simulink model "zynqRadioWalkieTalkieRxAD9361AD9364SL"  (R2016a)
settings: Solver=ode45  StartTime=0.0  StopTime=inf  RelTol=1e-3
PostLoadFcn:
  | sdrzWalkieTalkieRxParams = zynqRadioWalkieTalkeRxHelperAD9361AD9364SL_SimParams;
  | sdrzWalkieTalkieRxHelper_ModelParamsMask('applyParametersToModel');
InitFcn:
  | sdrzWalkieTalkieRxParams = zynqRadioWalkieTalkeRxHelperAD9361AD9364SL_SimParams;
  | sdrzWalkieTalkieRxHelper_ModelParamsMask('applyParametersToModel');
undefined symbols (not defined in the file or in its folder): F, fdesignblkfcn, gcbh
libraries: dspsnks4 x1, sdrzblksprivate x1, zc706fmc234_lib x1, dspmlti4 x1, commrfcorlib x1
CloseFcn:
  | clear sdrzWalkieTalkieRxParams GoertzelCoeffs
Description:
  | This model uses Simulink(R) to receive an FM signal from a suitable commercial walkie-talkie using SDR hardware with Analog Devices FMCOMMS2/3/4.
settings Model: SimulationMode=accelerator  Creator=The MathWorks, Inc.  LastModifiedBy=The MathWorks, Inc.
settings DataIOCC: LimitDataPoints=on  SaveFormat=Array
settings DebuggingCC: SolverPrmCheckMsg=warning  ParameterPrecisionLossMsg=none  AllowSymbolicDim=off
settings HardwareCC: ProdBitPerPointer=32  ProdLargestAtomicFloat=None  ProdIntDivRoundTo=Undefined  ProdEndianess=Unspecified  ProdWordSize=32  ProdHWDeviceType=32-bit Generic
settings ModelReferenceCC: PropagateSignalLabelsOutOfModel=off
settings ConfigComp: CovModelRefEnable=Off  CovSFcnEnable=off

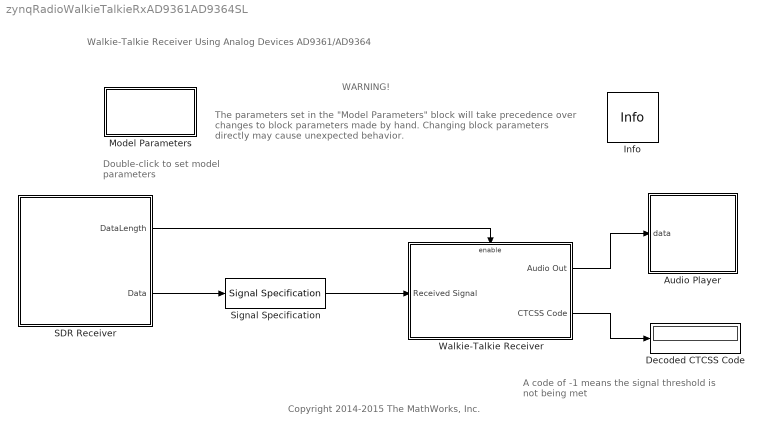
== system zynqRadioWalkieTalkieRxAD9361AD9364SL ==
  note: A code of -1 means the signal threshold
      | is not being met
  note: Walkie-Talkie Receiver Using Analog Devices AD9361/AD9364
  note: Double-click to
      | set model parameters
  note: The parameters set in the "Model Parameters" block will
      | take precedence over changes to block parameters made by hand.
      | Changing block parameters directly may cause unexpected behavior.
  note: WARNING!
  note: Copyright 2014-2015 The MathWorks, Inc.
  Audio Player : Subsystem
  Decoded CTCSS Code : Display
  Info : sdrzblksprivate/Info  SystemSampleTime=-1
  Model Parameters : Subsystem  TreatAsAtomicUnit=on  mask(Model Parameters){walkieTalkieProtocol=FRS, channelFRS=1, channelPMR446=4, CTCSSCode=5, CTCSSDecodeBlockLength=4000, signalPowerThreshold=0.1}
      mask prompts: walkieTalkieProtocol "Walkie-talkie protocol:"; channelFRS "Channel (1 to 14):"; channelPMR446 "Channel (1 to 8):"; CTCSSCode "CTCSS code (0 to 38):"; CTCSSDecodeBlockLength "CTCSS decode block length:"; signalPowerThreshold "Signal threshold for squelch:"
      mask help: Changing these values defines the model parameters needed for reception.
      mask init:
      | sdrzWalkieTalkieRxHelper_ModelParamsMask('applyParametersToModel');
      mask Help: sdrzdemohelp;
      mask TypeOptions walkieTalkieProtocol: FRS | PMR446
      mask Callback walkieTalkieProtocol: sdrzWalkieTalkieRxHelper_ModelParamsMask('maskDisplayUpdate');
      mask Display: disp('Model\nParameters');
  SDR Receiver : Subsystem
  Signal Specification : SignalSpecification  SampleTime=sdrzWalkieTalkieRxParams.radioFrameSize/sdrzWalkieTalkieRxParams.radioSampleRate
  Walkie-Talkie Receiver : Subsystem
  wires:
  Walkie-Talkie Receiver/2(CTCSS Code) -> Decoded CTCSS Code/1
  SDR Receiver/1(DataLength) -> Walkie-Talkie Receiver/Enable
  Walkie-Talkie Receiver/1(Audio Out) -> Audio Player/1(data)
  SDR Receiver/2(Data) -> Signal Specification/1
  Signal Specification/1 -> Walkie-Talkie Receiver/1(Received Signal)

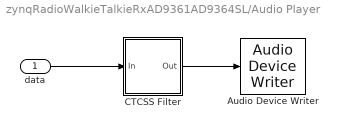
== system zynqRadioWalkieTalkieRxAD9361AD9364SL/Audio Player ==
  data : Inport
  Audio Device Writer : dspsnks4/Audio Device Writer  Driver=DirectSound  Device=Default  InheritSampleRate=off  SampleRate=8e3  BitDepth=16-bit integer  BufferSize=4096  NumBuffers=10  DefaultOutputChannelMapping=on  OutputChannelMapping=1:2  OutputNumUnderrunSamples=off  DriverIdx=1  DeviceWarnFlag=''
  CTCSS Filter : Subsystem  DialogController=fdesignblkfcn  InitFcn=fdesignblkfcn(gcbh, {'InitFcn'});  mask(Highpass Filter){}
      mask help: Design a highpass filter
      settings: CopyFcn=fdesignblkfcn(gcbh, {'CopyFcn'});
      mask Help: helpview(mapfilelocation('dsp'), 'dsphighpassfilter');
      mask Display: disp('Highpass')
  wires:
  data/1 -> CTCSS Filter/1(In)
  CTCSS Filter/1(Out) -> Audio Device Writer/1

== system zynqRadioWalkieTalkieRxAD9361AD9364SL/Model Parameters ==
  note: This subsystem is empty.
      | It is used for setting parameter values (in the mask).

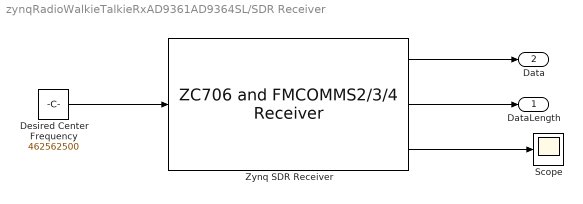
== system zynqRadioWalkieTalkieRxAD9361AD9364SL/SDR Receiver ==
  Desired Center Frequency : Constant  Value=462562500
  Scope : Scope
  Zynq SDR Receiver : zc706fmc234_lib/ZC706 and  FMCOMMS2//3//4  Receiver  IPAddress=192.168.3.2  CenterFrequencySource=Input port  CenterFrequency=2400000000  GainSource=AGC Fast Attack  Gain=1  ChannelMapping=1  BasebandSampleRate=sdrzWalkieTalkieRxParams.radioSampleRate  EnableBurstMode=off  NumFramesInBurst=20  OutputDataType=single  SamplesPerFrame=sdrzWalkieTalkieRxParams.radioFrameSize  LostSamplesOutputPort=on  RSSIOutputPort=off  DMATimeoutValue=1  blockMode=Normal  EnableQuadratureTracking=on  EnableRFDCTracking=on  EnableBasebandDCTracking=on  BypassUserLogic=on  ShowAdvancedProperties=on  ShowInternalProperties=off  subDeviceList=zynqReceiver  sdrExecutionMode=HW  dataUDPPort=-1  ctrlUDPPort=-1  SourceSelect=RF data  SourceConfiguration1=1023  FIRCoefficientSize=[ 128; 128 ]  FIRCoefficients=[ 111, -87, 147, -127, -18, -286, -312, -555, -601, -722, -642, -555, -303, -66, 221, 393, 488, 403, 219, -74, -343, -550, -582, -450, -146, 221, 569, 759, 735, 463, 20, -487, -885, -1048, -883, -418, 243, 897, 1340, 1394, 1002, 228, -715, -1549, -1980, -1819, -1028, 217, 1583, 2635, 2980, 2377, 853, -1275, -3435, -4926, -5080, -3454, 40, 5065, 10903, 16581, 21085, 23573, 23573, 21085, 16581, 10903, 5065, 40, -3454, -5080, -4926, -3435, -1275, 853, 2377, 2980, 2635, 1583, 217, -1028, -1819, -1980, -1549, -715, 228, 1002, 1394, 1340, 897, 243, -418, -883, -1048, -885, -487, 20, 463, 735, 759, 569, 221, -146, -450, -582, -550, -343, -74, 219, 403, 488, 393, 221, -66, -303, -555, -642, -722, -601, -555, -312, -286, -18, -127, 147, -87, 111; 382, -200, 711, -41, 645, 36, 346, -194, -119, -543, -472, -646, -404, -312, 45, 197, 413, 346, 241, -93, -373, -680, -755, -689, -356, 51, 515, 795, 870, 609, 136, -488, -1009, -1303, -1191, -712, 69, 885, 1516, 1692, 1336, 468, -662, -1740, -2378, -2329, -1494, -55, 1620, 2995, 3584, 3045, 1368, -1121, -3755, -5708, -6156, -4542, -710, 4969, 11669, 18243, 23486, 26391, 26391, 23486, 18243, 11669, 4969, -710, -4542, -6156, -5708, -3755, -1121, 1368, 3045, 3584, 2995, 1620, -55, -1494, -2329, -2378, -1740, -662, 468, 1336, 1692, 1516, 885, 69, -712, -1191, -1303, -1009, -488, 136, 609, 870, 795, 515, 51, -356, -689, -755, -680, -373, -93, 241, 346, 413, 197, 45, -312, -404, -646, -472, -543, -119, -194, 346, 36, 645, -41, 711, -200, 382 ]  FIRGain=[ 0; -12 ]  FIRDecimInterpFactor=[ 4; 4 ]  AnalogFilterCutoff=[ 2560000; 2560000 ]  FilterPathRates=[ 737280000, 184320000, 61440000, 30720000, 15360000, 3840000; 737280000, 184320000, 61440000, 30720000, 15360000, 3840000 ]  FilterDesignTypeForTx=DefaultFilterFromOther  FilterDesignTypeForRx=DefaultFilter  BISTLoopbackConfig=No Loopback  BISTPRBSMode=PRBS Disable  BISTToneMode=Tone Disable  BISTToneFrequency=F/32  BISTToneLevel=-6  BISTChannelMask=0  DataIsComplex=on  SimulateUsing=Code generation
  DataLength : Outport
  Data : Outport  Port=2
  wires:
  Desired Center Frequency/1 -> Zynq SDR Receiver/1
  Zynq SDR Receiver/1 -> Data/1
  Zynq SDR Receiver/2 -> DataLength/1
  Zynq SDR Receiver/3 -> Scope/1

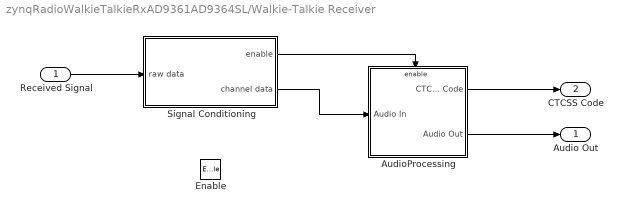
== system zynqRadioWalkieTalkieRxAD9361AD9364SL/Walkie-Talkie Receiver ==
  Received Signal : Inport
  Enable : EnablePort
  AudioProcessing : Subsystem
  Signal Conditioning : Subsystem
  Audio Out : Outport
  CTCSS Code : Outport  Port=2
  wires:
  AudioProcessing/1(CTCSS Code) -> CTCSS Code/1
  Received Signal/1 -> Signal Conditioning/1(raw data)
  Signal Conditioning/1(enable) -> AudioProcessing/Enable
  Signal Conditioning/2(channel data) -> AudioProcessing/1(Audio In)
  AudioProcessing/2(Audio Out) -> Audio Out/1

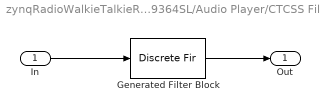
== system zynqRadioWalkieTalkieRxAD9361AD9364SL/Audio Player/CTCSS Filter ==
  In : Inport
  Generated Filter Block : DiscreteFir  Tag=BlockMethodSubSystem  Coefficients=[-0.028925555785371964 -1.1648489870143571e-05 0.00073703943806698632 0.002066323838223116 0.0037924562782123907 0.0058809478036791355 0.0081971633397573667 0.010595694447078679 0.012921336253850104 0.014980443784285901 0.016607828452391647 0.017600625095919989 0.017813808896053544 0.017076060612393459 0.015299380030688972 0.012382878571311963 0.0083283365848107558 0.0031334656085627169 -0.0030917556069984618 -0.010241846567876205 -0.018101550372905492 -0.026471631762265586 -0.035057392286144691 -0.043601476311625496 -0.051774176996057554 -0.059310312221053048 -0.065899215924792212 -0.071322316398364768 -0.075340335280439027 -0.07782838116556251 0.92134179186288967 -0.07782838116556251 -0.075340335280439027 -0.071322316398364768 -0.065899215924792212 -0.059310312221053048 -0.051774176996057554 -0.043601476311625496 -0.035057392286144691 -0.026471631762265586 -0.018101550372905492 -0.010241846567876205 -0.0030917556069984618 0.0031334656085627169 0.0083283365848107558 0.012382878571311963 0.015299380030688972 0.017076060612393459 0.017813808896053544 0.017600625095919989 0.016607828452391647 0.014980443784285901 0.012921336253850104 0.010595694447078679 0.0081971633397573667 0.0058809478036791355 0.0037924562782123907 0.002066323838223116 0.00073703943806698632 -1.1648489870143571e-05 -0.028925555785371964]  InputProcessing=Columns as channels (frame based)
  Out : Outport
  wires:
  In/1 -> Generated Filter Block/1
  Generated Filter Block/1 -> Out/1

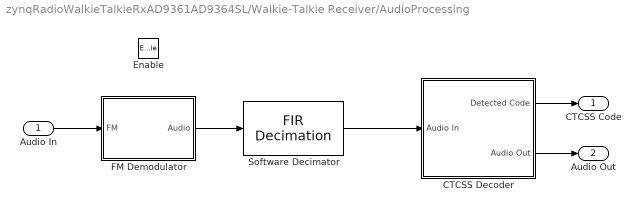
== system zynqRadioWalkieTalkieRxAD9361AD9364SL/Walkie-Talkie Receiver/AudioProcessing ==
  Audio In : Inport
  Enable : EnablePort
  CTCSS Decoder : Subsystem
  FM Demodulator : Subsystem
  Software Decimator : dspmlti4/FIR Decimation  FilterSource=Auto  h=sdrzWalkieTalkieRxParams.decimationCoefficients  D=sdrzWalkieTalkieRxParams.softwareDecimationFactor  filtStruct=Direct form  FilterObject=FDECIM  InputProcessing=Columns as channels (frame based)  framing=Enforce single-rate processing  inputOffset=0  outputBufInitCond=0  roundingMode=Floor  overflowMode=off  firstCoeffDataTypeStr=Inherit: Same word length as input  firstCoeffMin=[]  firstCoeffMax=[]  firstCoeffLastDataTypeStr=Inherit: Same word length as input  outputDataTypeStr=Inherit: Same as accumulator  outputMin=[]  outputMax=[]  outputLastDataTypeStr=Inherit: Same as accumulator
  CTCSS Code : Outport  OutputWhenDisabled=reset  InitialOutput=-1
  Audio Out : Outport  Port=2  OutputWhenDisabled=reset  InitialOutput=0
  wires:
  Software Decimator/1 -> CTCSS Decoder/1(Audio In)
  Audio In/1 -> FM Demodulator/1(FM)
  FM Demodulator/1(Audio) -> Software Decimator/1
  CTCSS Decoder/1(Detected Code) -> CTCSS Code/1
  CTCSS Decoder/2(Audio Out) -> Audio Out/1

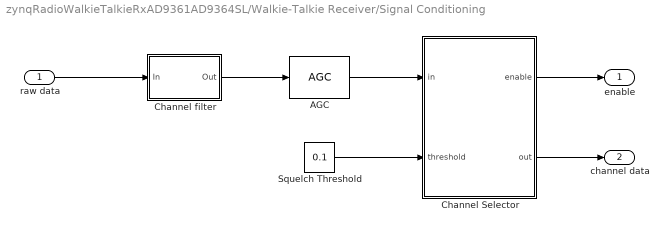
== system zynqRadioWalkieTalkieRxAD9361AD9364SL/Walkie-Talkie Receiver/Signal Conditioning ==
  raw data : Inport
  AGC : commrfcorlib/AGC  LegacyMode=off  DetectorMethod=Rectifier  LoopMethod=Linear  UpdatePeriod=200  StepSize=0.1  AdaptationStepSize=0.01  DesiredOutputPower=1  AveragingLength=100  MaximumGain=1e6  MaxPowerGain=60  GainOutputPort=off  InputPowerOutputPort=off  SimulateUsing=Code generation
  Channel Selector : MATLAB Function  TreatAsAtomicUnit=on
  Channel filter : Subsystem  DialogController=fdesignblkfcn  InitFcn=fdesignblkfcn(gcbh, {'InitFcn'});  mask(Lowpass Filter){}
      mask help: Design a lowpass filter
      settings: CopyFcn=fdesignblkfcn(gcbh, {'CopyFcn'});
      mask Help: helpview(mapfilelocation('dsp'), 'dsplowpassfilter');
      mask Display: disp('Lowpass')
  Squelch Threshold : Constant  Value=0.1  VectorParams1D=off  OutDataTypeStr=single  FramePeriod=-1
  enable : Outport
  channel data : Outport  Port=2
  wires:
  Squelch Threshold/1 -> Channel Selector/2(threshold)
  raw data/1 -> Channel filter/1(In)
  Channel Selector/2(out) -> channel data/1
  Channel Selector/1(enable) -> enable/1
  Channel filter/1(Out) -> AGC/1
  AGC/1 -> Channel Selector/1(in)

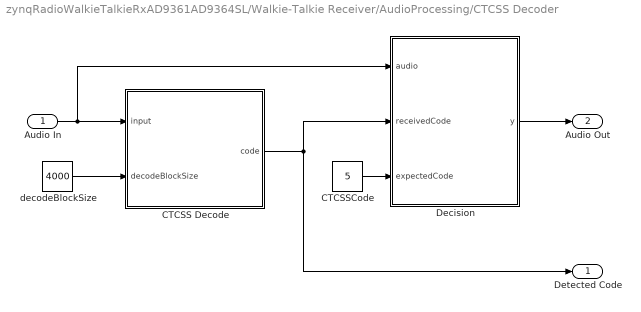
== system zynqRadioWalkieTalkieRxAD9361AD9364SL/Walkie-Talkie Receiver/AudioProcessing/CTCSS Decoder ==
  Audio In : Inport
  CTCSS Decode : MATLAB Function  TreatAsAtomicUnit=on
  CTCSSCode : Constant  Value=5
  Decision : MATLAB Function  TreatAsAtomicUnit=on
  decodeBlockSize : Constant  Value=4000
  Detected Code : Outport
  Audio Out : Outport  Port=2
  wires:
  CTCSSCode/1 -> Decision/3(expectedCode)
  Audio In/1 -> Decision/1(audio), CTCSS Decode/1(input)
  CTCSS Decode/1(code) -> Decision/2(receivedCode), Detected Code/1
  Decision/1(y) -> Audio Out/1
  decodeBlockSize/1 -> CTCSS Decode/2(decodeBlockSize)

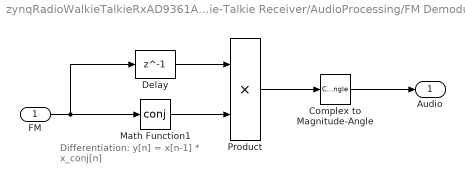
== system zynqRadioWalkieTalkieRxAD9361AD9364SL/Walkie-Talkie Receiver/AudioProcessing/FM Demodulator ==
  note: Differentiation:
      | y[n] = x[n-1] * x_conj[n]
  FM : Inport
  Complex to Magnitude-Angle : ComplexToMagnitudeAngle  Output=Angle
  Delay : Delay  DelayLength=1  InitialCondition=0  InputProcessing=Columns as channels (frame based)
  Math Function1 : Math  Operator=conj  SaturateOnIntegerOverflow=on
  Product : Product  RndMeth=Zero
  Audio : Outport
  wires:
  Complex to Magnitude-Angle/1 -> Audio/1
  Math Function1/1 -> Product/2
  FM/1 -> Math Function1/1, Delay/1
  Delay/1 -> Product/1
  Product/1 -> Complex to Magnitude-Angle/1

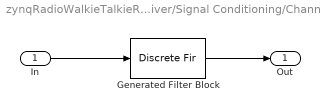
== system zynqRadioWalkieTalkieRxAD9361AD9364SL/Walkie-Talkie Receiver/Signal Conditioning/Channel filter ==
  In : Inport
  Generated Filter Block : DiscreteFir  Tag=BlockMethodSubSystem  FilterStructure=Direct form transposed  Coefficients=[-0.12615211506985044 0.054435505076490753 0.046014523279817872 0.040714483430476123 0.037234012875121465 0.035093626124781854 0.034279118732135891 0.033944271562873655 0.034436407356210834 0.035132040956212647 0.036213537898985543 0.037335073385194081 0.038531318224554516 0.039680613168755881 0.040760846004675021 0.041745545861175112 0.042616680139951325 0.043324412723859146 0.043889922453143354 0.044205914318413406 0.044351496210509378 0.044205914318413406 0.043889922453143354 0.043324412723859146 0.042616680139951325 0.041745545861175112 0.040760846004675021 0.039680613168755881 0.038531318224554516 0.037335073385194081 0.036213537898985543 0.035132040956212647 0.034436407356210834 0.033944271562873655 0.034279118732135891 0.035093626124781854 0.037234012875121465 0.040714483430476123 0.046014523279817872 0.054435505076490753 -0.12615211506985044]  InputProcessing=Columns as channels (frame based)
  Out : Outport
  wires:
  In/1 -> Generated Filter Block/1
  Generated Filter Block/1 -> Out/1

== matlab function zynqRadioWalkieTalkieRxAD9361AD9364SL/Walkie-Talkie Receiver/Signal Conditioning/Channel Selector ==
  data: in input; enable output; threshold input; out output size=[sdrzWalkieTalkieRxParams.radioFrameSize, 1]
function [enable, out] = squelchFilter(in, threshold)
%#codegen
% Compute the average power of the input signal, if it is greater than a
% threshold, set the enable high, otherwise, low.
out = in;

len = length(in); 
power = sum(abs(in)) / len;

if (power >= threshold)
    enable = true;
else 
    enable = false;
end

== matlab function zynqRadioWalkieTalkieRxAD9361AD9364SL/Walkie-Talkie Receiver/AudioProcessing/CTCSS Decoder/Decision ==
  data: audio input; y output size=[sdrzWalkieTalkieRxParams.radioFrameSize/sdrzWalkieTalkieRxParams.softwareDecimationFactor, 1]; receivedCode input; expectedCode input
function y  = CTCSSCodeCompare(audio, receivedCode, expectedCode)
%#codegen

% If the decoded code equals to pre-specified code, or the pre-specified
% code is 0 (no CTCSS), the audio signal goes through, otherwise, output
% zero.

if ((receivedCode == expectedCode) || (expectedCode == 0))
    y = audio;
else
    y = single(zeros(length(audio),1));
end

== matlab function zynqRadioWalkieTalkieRxAD9361AD9364SL/Walkie-Talkie Receiver/AudioProcessing/CTCSS Decoder/CTCSS Decode ==
  data: input input; code output int8; GoertzelCoeffs parameter; decodeBlockSize input
function code  = CTCSS_Decode(input, GoertzelCoeffs, decodeBlockSize)
%#codegen
% CTCSS decoder for use in a tone squelch system.
%
% Requires identification of one of a set of tones in the audio stream.
% Input is a frame of audio samples at a sample rate of (close to) 8kHz.
%
% Each time the function is called when a frame of samples comes in. It
% changes the state of the function, s(n), s(n-1), s(n-2). When a block of
% samples passes through (block size specified by frs_decodeBlockSize ),
% the power at each frequency is computed by Goertzel algorithm and the
% state is cleared to zero, preparing for the next block. The block size
% could be much larger than the frame size. 
%
% Below is the frequency table for private codes. 
% 
% PL   Hz     PL   Hz      PL   Hz
% --  ----    --  -----    --  -----
%  1  67.0    12  100.0    32  203.5
%  2  71.9    13  103.5    33  210.7
%  3  74.4    14  107.2    34  218.1
%  4  77.0    15  110.9    35  225.7
%  5  79.7    16  114.8    36  233.6
%  6  82.5    17  118.8    37  241.8
%  7  85.4    18  123.0    38  250.3
%  8  88.5    19  127.3
%  9  91.5    20  131.8
% 10  94.8    21  136.5
% 11  97.4    22  141.3
%             23  146.2
%             24  151.4
%             25  156.7
%             26  162.2
%             27  167.9
%             28  173.8
%             29  179.9
%             30  186.2
%             31  192.8
 
nTones = length(GoertzelCoeffs);

persistent  s_d1 s_d2 s maxPowerIdx nProcessed

if isempty(s_d1)
    s_d1 = coder.nullcopy(single(zeros(nTones,1)));% s_d1 = s(n-1)
    s_d2 = coder.nullcopy(single(zeros(nTones,1)));% s_d2 = s(n-2)
    s = coder.nullcopy(single(zeros(nTones,1))); % s = s(n)
    nProcessed = 0;
    maxPowerIdx = 0; 
end

frameSize = length(input);

% The number of sample needs to be processed
nSampleProc = min(frameSize, decodeBlockSize - nProcessed);

for i = 1:nSampleProc
	inputVec = repmat(input(i), nTones,1);
    % s(n) = x(n) + 2cos(2*pi*w)s(n-1) - s(n-2)
	s  = inputVec + GoertzelCoeffs .* s_d1 - s_d2; 
	s_d2 = s_d1;
	s_d1 = s;
end

nProcessed  = nProcessed + nSampleProc;

% if a block is done
if (nProcessed == decodeBlockSize)
	
	power = s_d2.^2 + s_d1.^2 - GoertzelCoeffs .* s_d2 .* s_d1;

    if (any(power ~= 0))
        [~, maxPowerIdx] = max(power);
    end

    % clear the state
	s_d1 = single(zeros(nTones,1));
	s_d2 = single(zeros(nTones,1));
	
    % next block starts, process the remaining samples in the current frame
	for i = nSampleProc + 1 : frameSize
		inputVec = repmat(input(i), nTones,1);
		s  = inputVec + GoertzelCoeffs .* s_d1 - s_d2;
		s_d2 = s_d1;
		s_d1 = s;
	end
	nProcessed = frameSize - nSampleProc;

end

code = int8(maxPowerIdx);
